simulink model "Subsystem"  (R2020a)
settings: Solver=FixedStepAuto  StartTime=0.0  StopTime=10.0  FixedStep=0.2  RelTol=1e-3
settings Model: Creator=Viraj  LastModifiedBy=Viraj
settings DataIOCC: SaveOutput=off  SaveTime=off

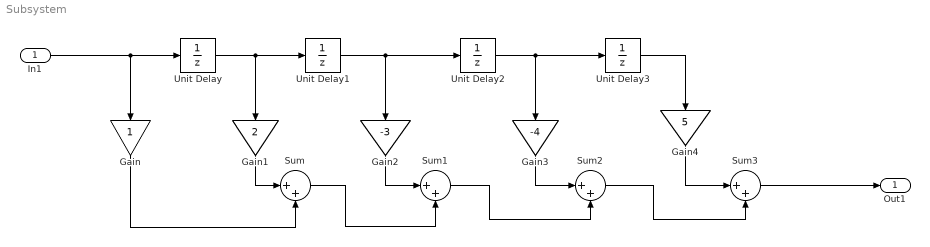
== system Subsystem ==
  In1 : Inport  OutDataTypeStr=double  PortDimensions=1  SampleTime=[0.20000000000000001,0]
  Gain : Gain
  Gain1 : Gain  Gain=2
  Gain2 : Gain  Gain=-3
  Gain3 : Gain  Gain=-4
  Gain4 : Gain  Gain=5
  Sum{,1..3} (4 alike) : Sum  Inputs=|++
  Unit Delay{,1..3} (4 alike) : UnitDelay  SampleTime=-1  HasFrameUpgradeWarning=on
  Out1 : Outport  OutDataTypeStr=double  PortDimensions=1  SampleTime=[0.20000000000000001,0]
  wires:
  Sum/1 -> Sum1/2
  Sum1/1 -> Sum2/2
  Gain2/1 -> Sum1/1
  Unit Delay/1 -> Gain1/1, Unit Delay1/1
  Gain1/1 -> Sum/1
  Gain3/1 -> Sum2/1
  Gain/1 -> Sum/2
  Unit Delay1/1 -> Gain2/1, Unit Delay2/1
  Unit Delay3/1 -> Gain4/1
  Unit Delay2/1 -> Gain3/1, Unit Delay3/1
  In1/1 -> Gain/1, Unit Delay/1
  Gain4/1 -> Sum3/1
  Sum2/1 -> Sum3/2
  Sum3/1 -> Out1/1
